simulink library "ESTS_REV"  (R2024b)
settings: Solver=VariableStepAuto  StartTime=0.0  StopTime=10.0  RelTol=1e-3
undefined symbols (not defined in the file or in its folder): p_dt_s, p_Ests_Rev_MaxA_mps2, p_RadWhlDynFr_m, p_RadWhlDynRe_m, p_trackFr_m, p_trackRe_m
settings Model: Creator=blatak  LastModifiedBy=blatak
settings ModelReferenceCC: EnableRefExpFcnMdlSchedulingChecks=on
settings RTWCC: GPUComputeCapability=3.5

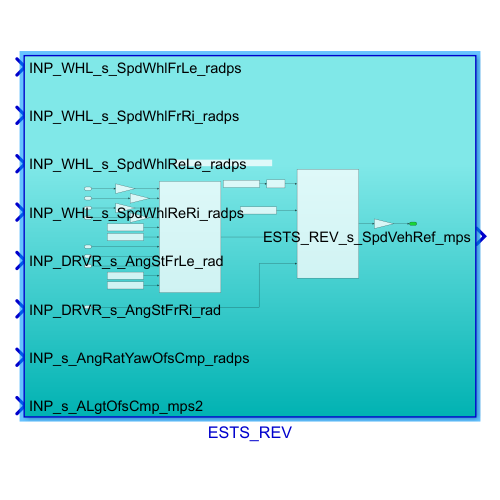
[thumbnail: Simulink's stored preview of the top-level diagram]
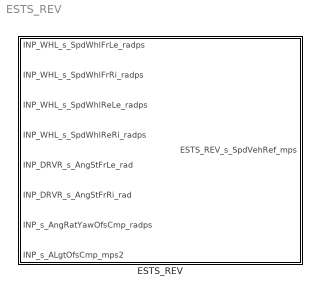
== system ESTS_REV ==
  ESTS_REV : Subsystem

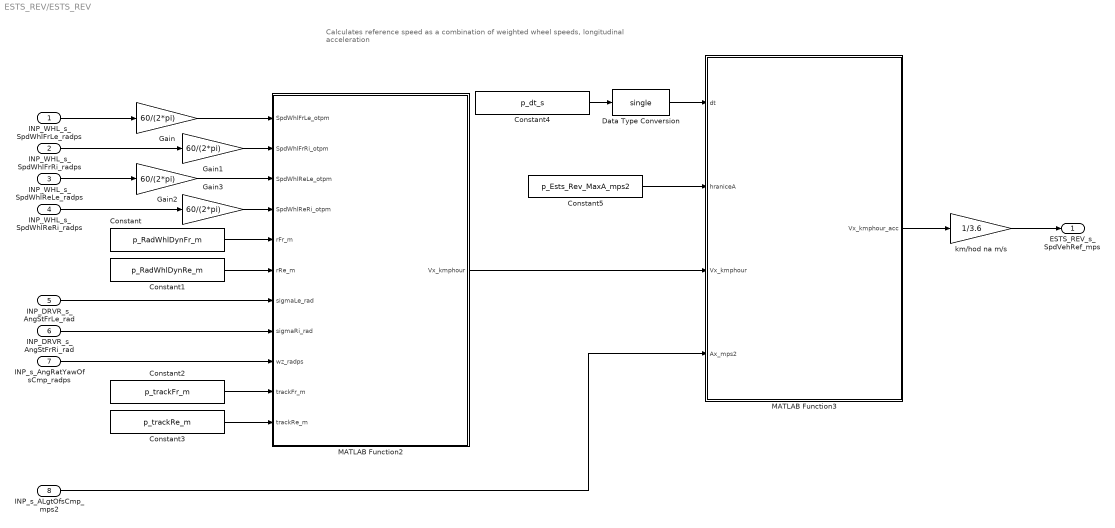
== system ESTS_REV/ESTS_REV ==
  note: Calculates reference speed as a combination of weighted wheel speeds, longitudinal acceleration
  INP_WHL_s_SpdWhlFrLe_radps : Inport
  INP_WHL_s_SpdWhlFrRi_radps : Inport  Port=2
  INP_WHL_s_SpdWhlReLe_radps : Inport  Port=3
  INP_WHL_s_SpdWhlReRi_radps : Inport  Port=4
  INP_DRVR_s_AngStFrLe_rad : Inport  Port=5
  INP_DRVR_s_AngStFrRi_rad : Inport  Port=6
  INP_s_AngRatYawOfsCmp_radps : Inport  Port=7
  INP_s_ALgtOfsCmp_mps2 : Inport  Port=8
  Constant : Constant  Value=p_RadWhlDynFr_m
  Constant1 : Constant  Value=p_RadWhlDynRe_m
  Constant2 : Constant  Value=p_trackFr_m
  Constant3 : Constant  Value=p_trackRe_m
  Constant4 : Constant  Value=p_dt_s
  Constant5 : Constant  Value=p_Ests_Rev_MaxA_mps2
  Data Type Conversion : DataTypeConversion  OutDataTypeStr=single  SaturateOnIntegerOverflow=off  RndMeth=Floor
  Gain{,1..3} (4 alike) : Gain  Gain=60/(2*pi)
  MATLAB Function2 : MATLAB Function  TreatAsAtomicUnit=on
  MATLAB Function3 : MATLAB Function  TreatAsAtomicUnit=on
  km/hod na m/s : Gain  Gain=1/3.6
  ESTS_REV_s_SpdVehRef_mps : Outport
  wires:
  INP_WHL_s_SpdWhlReRi_radps/1 -> Gain3/1
  INP_DRVR_s_AngStFrRi_rad/1 -> MATLAB Function2/8(sigmaRi_rad)
  Constant5/1 -> MATLAB Function3/2(hraniceA)
  Constant2/1 -> MATLAB Function2/10(trackFr_m)
  Gain1/1 -> MATLAB Function2/2(SpdWhlFrRi_otpm)
  INP_WHL_s_SpdWhlReLe_radps/1 -> Gain2/1
  Gain/1 -> MATLAB Function2/1(SpdWhlFrLe_otpm)
  MATLAB Function3/1(Vx_kmphour_acc) -> km/hod na m/s/1
  Constant3/1 -> MATLAB Function2/11(trackRe_m)
  km/hod na m/s/1 -> ESTS_REV_s_SpdVehRef_mps/1
  INP_s_ALgtOfsCmp_mps2/1 -> MATLAB Function3/4(Ax_mps2)
  Constant/1 -> MATLAB Function2/5(rFr_m)
  Gain2/1 -> MATLAB Function2/3(SpdWhlReLe_otpm)
  INP_DRVR_s_AngStFrLe_rad/1 -> MATLAB Function2/7(sigmaLe_rad)
  Constant1/1 -> MATLAB Function2/6(rRe_m)
  MATLAB Function2/1(Vx_kmphour) -> MATLAB Function3/3(Vx_kmphour)
  INP_s_AngRatYawOfsCmp_radps/1 -> MATLAB Function2/9(wz_radps)
  Constant4/1 -> Data Type Conversion/1
  Gain3/1 -> MATLAB Function2/4(SpdWhlReRi_otpm)
  INP_WHL_s_SpdWhlFrRi_radps/1 -> Gain1/1
  INP_WHL_s_SpdWhlFrLe_radps/1 -> Gain/1
  Data Type Conversion/1 -> MATLAB Function3/1(dt)

== matlab function ESTS_REV/MATLAB Function3 ==
  data: dt input; Vx_kmphour_acc output; hraniceA input; Vx_kmphour input; Ax_mps2 input
function Vx_kmphour_acc = fce_Vx_Rpm_Acc(dt, hraniceA, Vx_kmphour, Ax_mps2)
% Funkce vahuje dva zdroje Vx a to z kol a ze zrychleni na zaklade
% velikosti Ax
% Pokud se neveri kolum, vice se veri prirustku ze zrychleni
% Ax - Ax v g
% Vx_rpm - Rychlost odhadovana z otacek kol
% hraniceA - hranice, ke ktere se prepocitava pomer /pro bela to bylo 0,57g
% Fvz - pro vypocet dT protoze se prirustkove integruje

persistent Vx_rpm_acc_prev
if isempty(Vx_rpm_acc_prev)
    Vx_rpm_acc_prev = single(0);
end

maxA = hraniceA;

prcA = abs(Ax_mps2)/(maxA/100);

if prcA > 100
    prcA = single(100);
end

prcRPM = 100-prcA;

dV = (Ax_mps2*dt)*3.6;

Vx_kmphour_acc = (prcA/100)*(Vx_rpm_acc_prev + dV) + (prcRPM/100)*Vx_kmphour;

Vx_rpm_acc_prev = Vx_kmphour_acc;

== matlab function ESTS_REV/MATLAB Function2 ==
  data: SpdWhlFrLe_otpm input; Vx_kmphour output; SpdWhlFrRi_otpm input; SpdWhlReLe_otpm input; SpdWhlReRi_otpm input; rFr_m input; rRe_m input; sigmaLe_rad input; sigmaRi_rad input; wz_radps input; trackFr_m input; trackRe_m input
function Vx_kmphour = fce_Vx_Rpm_GeomMean(SpdWhlFrLe_otpm, SpdWhlFrRi_otpm, SpdWhlReLe_otpm, SpdWhlReRi_otpm, rFr_m, rRe_m, sigmaLe_rad, sigmaRi_rad, wz_radps, trackFr_m, trackRe_m)
% rpmFL, rpmFR, rpmRL, rpmRR - otacky kol za minutu
% rF, rR - polomery kol predni a zadni [m]
% sigmaL, sigmaR - natoceni kol [radiany]
% wz - uhlova rychlost v ose Z [radiany]
% trackF, trackR - rozchod kol [m]

% obvod kol
oF=2*pi*rFr_m;
oR=2*pi*rRe_m;

% merena rychlost kol km/h
speedMeasFL=(SpdWhlFrLe_otpm*60)*(oF/1000);
speedMeasFR=(SpdWhlFrRi_otpm*60)*(oF/1000);
speedMeasRL=(SpdWhlReLe_otpm*60)*(oR/1000);
speedMeasRR=(SpdWhlReRi_otpm*60)*(oR/1000);

% prepocet delky z metru na km
LF=trackFr_m/1000;
LR=trackRe_m/1000;

% rychlosti jednotlivých kol
speedFL = speedMeasFL * cos(sigmaLe_rad) - wz_radps * (LF/2); % predni kola se nataci
speedFR = speedMeasFR * cos(sigmaRi_rad) + wz_radps * (LF/2); % predni kola se nataci
speedRL = speedMeasRL - wz_radps * (LR/2); % zadni kola jsou pevna
speedRR = speedMeasRR + wz_radps * (LR/2); % zadni kola jsou pevna

% rychlost Vx
Vx_kmphour = mean([speedFL, speedFR, speedRL, speedRR]);
